simulink model "model4"  (R2024b)
settings: Solver=FixedStepAuto  StartTime=0.0  StopTime=500  FixedStep=0.001  RelTol=1e-3  EnableMultiTasking=on
libraries: arduinolib x2
settings Model: ExtModeTrigDuration=2  Creator=USER  LastModifiedBy=USER
settings SolverCC: AutoInsertRateTranBlk=on
settings OptimizationCC: EnhancedBackFolding=on  PassReuseOutputArgsAs=Individual arguments  ZeroExternalMemoryAtStartup=off  ZeroInternalMemoryAtStartup=off  MaxStackSize=64  OptimizeBlockOrder=speed  DifferentSizesBufferReuse=on  OptimizationCustomize=off  EfficientTunableParamExpr=on
settings DebuggingCC: ParameterTunabilityLossMsg=error
settings HardwareCC: ProdBitPerInt=16  ProdBitPerPointer=16  ProdBitPerSizeT=16  ProdBitPerPtrDiffT=16  ProdLargestAtomicFloat=None  ProdWordSize=8  ProdHWDeviceType=Atmel->AVR
settings SFSimCC: MATLABDynamicMemAlloc=off
settings RTWCC: Description=Embedded Coder  SystemTargetFile=ert.tlc  HardwareBoard=Arduino Mega 2560  TemplateMakefile=ert_default_tmf  Toolchain=Arduino AVR  BuildConfiguration=Faster Runs
settings CodeAppCC: ForceParamTrailComments=on  IgnoreCustomStorageClasses=off  OperatorAnnotations=on  SimulinkDataObjDesc=on  SFDataObjDesc=on  InsertBlockDesc=on
settings ERTTargetCC: SupportContinuousTime=on  SupportVariableSizeSignals=on  ExtModeTransport=3  ExtModeStaticAlloc=on  ExtModeAutomaticAllocSize=off  ExtModeStaticAllocSize=2048  ExtModeMexFile=ext_xcp  ExtModeIntrfLevel=Level2 - Open  InlinedParameterPlacement=Hierarchical

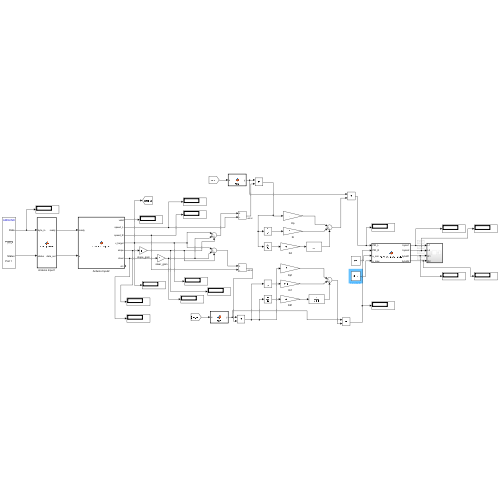
[thumbnail: Simulink's stored preview of the top-level diagram]
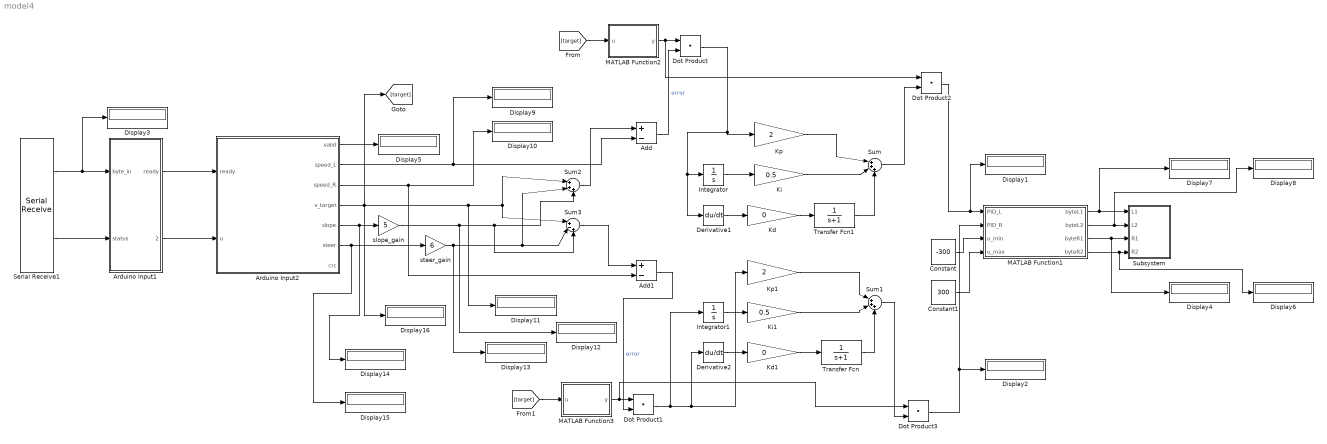
== system model4 ==
  Add : Sum  Inputs=+-  OutDataTypeStr=double  AccumDataTypeStr=double
  Add1 : Sum  Inputs=+-  OutDataTypeStr=double  AccumDataTypeStr=double
  Arduino Input1 : MATLAB Function  TreatAsAtomicUnit=on
  Arduino Input2 : MATLAB Function  TreatAsAtomicUnit=on
  Constant : Constant  Value=-300
  Constant1 : Constant  Value=300
  Derivative1 : Derivative
  Derivative2 : Derivative
  Display{1..16} (16 alike) : Display
      Display1 settings: Format=decimal (Stored Integer)
      Display10 settings: Format=decimal (Stored Integer)
      Display11 settings: Format=decimal (Stored Integer)
      Display13 settings: Format=decimal (Stored Integer)
      Display14 settings: Format=decimal (Stored Integer)
      Display15 settings: Format=decimal (Stored Integer)
      Display16 settings: Format=decimal (Stored Integer)
      Display2 settings: Format=decimal (Stored Integer)
      Display3 settings: Format=decimal (Stored Integer)
      Display4 settings: Format=decimal (Stored Integer)
      Display5 settings: Format=decimal (Stored Integer)
      Display6 settings: Format=decimal (Stored Integer)
      Display7 settings: Format=decimal (Stored Integer)
      Display8 settings: Format=decimal (Stored Integer)
      Display9 settings: Format=decimal (Stored Integer)
  Dot Product : DotProduct  OutDataTypeStr=Inherit: Inherit via internal rule
  Dot Product1 : DotProduct  OutDataTypeStr=Inherit: Inherit via internal rule
  Dot Product2 : DotProduct  OutDataTypeStr=int16
  Dot Product3 : DotProduct  OutDataTypeStr=int16
  Integrator : Integrator
  Integrator1 : Integrator
  Kd : Gain  Gain=0  ParamDataTypeStr=double  OutDataTypeStr=double
  Kd1 : Gain  Gain=0  ParamDataTypeStr=double  OutDataTypeStr=double
  Ki : Gain  Gain=0.5  ParamDataTypeStr=double  OutDataTypeStr=double
  Ki1 : Gain  Gain=0.5  ParamDataTypeStr=double  OutDataTypeStr=double
  Kp : Gain  Gain=2  ParamDataTypeStr=double  OutDataTypeStr=double
  Kp1 : Gain  Gain=2  ParamDataTypeStr=double  OutDataTypeStr=double
  MATLAB Function1 : MATLAB Function  TreatAsAtomicUnit=on
  MATLAB Function2 : MATLAB Function  TreatAsAtomicUnit=on
  MATLAB Function3 : MATLAB Function  TreatAsAtomicUnit=on
  Serial Receive1 : arduinolib/Serial Receive  portNumber=1  DataType=uint8  blockPlatform=ARDUINO  TimeOut=0  MaxDataLength=10  isARMArch=off  DataLengthOption=Length via dialog  Datalength=1  Header=[]  Terminator=[]  SampleTime=0.001  ShowOutStatus=on
      settings: SourceProductName=Common
  Subsystem : Subsystem  TreatAsAtomicUnit=on  SystemSampleTime=0.1
  Sum : Sum  Inputs=|+++  OutDataTypeStr=double
  Sum1 : Sum  Inputs=|+++  OutDataTypeStr=double
  Sum2 : Sum  Inputs=|+++  OutDataTypeStr=double  AccumDataTypeStr=double
  Sum3 : Sum  Inputs=|+-+  OutDataTypeStr=double  AccumDataTypeStr=double
  Transfer Fcn : TransferFcn  Denominator=[1 1]
  Transfer Fcn1 : TransferFcn  Denominator=[1 1]
  slope_gain : Gain  Gain=5
  steer_gain : Gain  Gain=6  ParamDataTypeStr=double  OutDataTypeStr=double
  wires:
  Arduino Input2/2(speed_L) -> Display9/1, Add/2
  Arduino Input2/4(v_target) -> [target], Display16/1, Display11/1, Sum2/1, Sum3/1
  Integrator/1 -> Ki/1
  Derivative1/1 -> Kd/1
  Kp/1 -> Sum/1
  Ki/1 -> Sum/2
  Kd/1 -> Transfer Fcn1/1
  Sum1/1 -> Dot Product3/2
  Arduino Input1/1(ready) -> Arduino Input2/1(ready)
  Serial Receive1/2 -> Arduino Input1/2(status)
  Arduino Input1/2(data_out) -> Arduino Input2/2(u)
  Serial Receive1/1 -> Display3/1, Arduino Input1/1(byte_in)
  Arduino Input2/3(speed_R) -> Add1/2, Display10/1
  Arduino Input2/1(valid) -> Display5/1
  Arduino Input2/6(steer) -> Display15/1, steer_gain/1
  steer_gain/1 -> Display13/1, Sum2/2, Sum3/2
  Sum2/1 -> Add/1
  Sum3/1 -> Add1/1
  Kd1/1 -> Transfer Fcn/1
  Ki1/1 -> Sum1/2
  Kp1/1 -> Sum1/1
  Derivative2/1 -> Kd1/1
  Integrator1/1 -> Ki1/1
  MATLAB Function1/2(byteL2) -> Display8/1, Subsystem/2(L2)
  MATLAB Function1/3(byteR1) -> Display4/1, Subsystem/3(R1)
  MATLAB Function1/4(byteR2) -> Display6/1, Subsystem/4(R2)
  Arduino Input2/5(slope) -> Display14/1, slope_gain/1
  slope_gain/1 -> Display12/1, Sum3/3, Sum2/3
  Transfer Fcn/1 -> Sum1/3
  Transfer Fcn1/1 -> Sum/3
  Sum/1 -> Dot Product2/2
  Constant/1 -> MATLAB Function1/3(u_min)
  Constant1/1 -> MATLAB Function1/4(u_max)
  MATLAB Function1/1(byteL1) -> Display7/1, Subsystem/1(L1)
  [target] -> MATLAB Function2/1(u)
  [target] -> MATLAB Function3/1(u)
  Add/1 -> Dot Product/2  "error"
  Dot Product/1 -> Derivative1/1, Integrator/1, Kp/1
  Add1/1 -> Dot Product1/2  "error"
  Dot Product1/1 -> Integrator1/1, Derivative2/1, Kp1/1
  MATLAB Function2/1(y) -> Dot Product2/1, Dot Product/1
  MATLAB Function3/1(y) -> Dot Product3/1, Dot Product1/1
  Dot Product3/1 -> MATLAB Function1/2(PID_R), Display2/1
  Dot Product2/1 -> Display1/1, MATLAB Function1/1(PID_L)

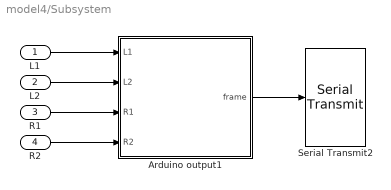
== system model4/Subsystem ==
  L1 : Inport
  L2 : Inport  Port=2
  R1 : Inport  Port=3
  R2 : Inport  Port=4
  Arduino output1 : MATLAB Function  TreatAsAtomicUnit=on
  Serial Transmit2 : arduinolib/Serial Transmit  portNumber=1  sendmode=write  sendformat=Decimal  floatprecision=2  header=[0xAA]  terminator=[0x55]  blockPlatform=ARDUINO
      settings: SourceProductName=Common
  wires:
  L2/1 -> Arduino output1/2(L2)
  Arduino output1/1(frame) -> Serial Transmit2/1
  L1/1 -> Arduino output1/1(L1)
  R1/1 -> Arduino output1/3(R1)
  R2/1 -> Arduino output1/4(R2)

== matlab function model4/MATLAB Function1 ==
  data: PID_L input; byteL1 output uint8; PID_R input; u_min input; u_max input; byteL2 output uint8; byteR1 output uint8; byteR2 output uint8
function [byteL1, byteL2, byteR1, byteR2] = encode_pwm_duty(PID_L, PID_R, u_min, u_max)
%#codegen

% [-1000, 1000] 범위로 선형 매핑
scale = 1000 / (u_max - u_min);
dutyL = int16(round((PID_L - u_min) * scale - 500));
dutyR = int16(round((PID_R - u_min) * scale - 500));

% uint16로 안전 변환 (비트 연산 위해)
dutyL_u = uint16(typecast(dutyL, 'uint16'));
dutyL_u = dutyL_u(1);
dutyR_u = uint16(typecast(dutyR, 'uint16'));
dutyR_u = dutyR_u(1);
% MSB / LSB 분리
byteL1 = uint8(bitshift(dutyL_u, -8));  % MSB
byteL2 = uint8(bitand(dutyL_u, 255));   % LSB

byteR1 = uint8(bitshift(dutyR_u, -8));
byteR2 = uint8(bitand(dutyR_u, 255));

% function [byteL1, byteL2, byteR1, byteR2] = encode_pwm_duty(PID_L, PID_R, u_min, u_max)
% % PID_L, PID_R : PID 제어기 출력값 (실수형)
% % u_min, u_max : PID 출력 예상 범위 (예: -4050 ~ +4050)
% 
% % 매핑 대상 범위
% min_duty = -1000;
% max_duty = 1000;
% 
% %% 매핑 함수 정의
% map_to_range = @(u) ((u - u_min) / (u_max - u_min)) * (max_duty - min_duty) + min_duty;
% 
% % 매핑 수행
% dutyL = int16(round(map_to_range(PID_L)));  % 정수로 변환
% dutyR = int16(round(map_to_range(PID_R)));
% 
% % MSB/LSB 분리
% byteL2 = bitand(dutyL, 255);         % LSB
% byteL1 = bitshift(dutyL, -8);        % MSB
% 
% byteR2 = bitand(dutyR, 255);
% byteR1 = bitshift(dutyR, -8);

== matlab function model4/MATLAB Function2 ==
  data: u input; y output
function y = fcn(u)

if u<1 && u > -1
    y=0;
else
    y=1;
end

== matlab function model4/Arduino Input2 ==
  data: ready input; valid output; speed_L output; speed_R output; v_target output; u input; slope output; steer output; crc output
function [valid, speed_L, speed_R, v_target, slope, steer, crc] =  Arduino_Input2( ready, u)
% UART 패킷 파서 (persistent 방식으로 이전 값 유지)
% u: [10x1] uint8, 패킷 데이터
% ready: 패킷 유효 신호

%#codegen

% 이전 출력값 저장용 persistent 변수
persistent p_valid p_speed_L p_speed_R p_v_target p_slope p_steer p_crc
 
% 초기화 (최초 실행 시)
if isempty(p_valid)
    p_valid = false;
    p_speed_L = 0.0;
    p_speed_R = 0.0;
    p_v_target = uint16(0);
    p_slope = int8(0);
    p_steer = int8(0);
    p_crc = uint8(0);
end

% 새로운 데이터가 들어왔을 경우만 업데이트
if ready == 1
    % data_sum = uint16((2)) + uint16(u(3)) + uint16(u(4)) + uint16(u(5)) + uint16(u(6)) + uint16(u(7)) + uint16(u(8)) + uint16(u(9));
    % if (0xFF & data_sum) == 0
        p_valid = true;
        p_speed_L = (double(u(2)-1) + double(u(3)-1)/100)*10;
        p_speed_R = (double(u(4)-1) + double(u(5)-1)/100)*10;
        if u(7)==1
            u(7)=u(7)-1;
        end
        p_v_target = uint16(u(7)-1)*10;
        tmp = typecast(u(6), 'int8'); tmp = tmp(1);
        if tmp <= int8(30) && tmp >= int8(-30)
            p_slope = tmp;
        end
        tmp = typecast(u(8), 'int8'); tmp = tmp(1);
        if  tmp <= int8(30) && tmp >= int8(-30)
            p_steer = tmp;
        end
        p_crc = u(9);
    % end
end

% 항상 마지막 유효 출력 반환
valid     = p_valid;
speed_L   = p_speed_L;
speed_R   = p_speed_R;
v_target  = p_v_target;
slope     = p_slope;
steer     = p_steer;
crc       = p_crc;

== matlab function model4/Arduino Input1 ==
  data: ready output; data_out output; byte_in input; status input
function [ready, data_out] = uart_parser(byte_in, status)
% UART 프레임 수신기 (Start Byte = 0xAA, Total = 10 bytes)
% 입력: byte_in - 1바이트씩 들어오는 uint8
% 입력: status - Serial Receive의 상태 (1이면 수신 성공)
% 출력: ready - 1이면 패킷 파싱 완료
% 출력: data_out - [1x10] uint8, 패킷 데이터

persistent buffer count collecting

if isempty(buffer)
    buffer = zeros(1, 10, 'uint8');
    count = 0;
    collecting = false;
end

ready = false;
data_out = zeros(1,10,'uint8');

if status == 1
    if ~collecting
        % 아직 수집 시작 전 → start byte 찾기
        if byte_in == hex2dec('AA')
            buffer(1) = byte_in;
            count = 1;
            collecting = true;
        end
    else
        if byte_in == hex2dec('AA')
            count = 1;
        end
        % 수집 중
        count = count + 1;
        buffer(count) = byte_in;

        if count == 10
            data_out = buffer;
            ready = true;
            count = 0;
            collecting = false;
        end
    end
else
    % if count~=0
    %     count = count + 1;
    %     buffer(count) = uint8(0);
    %     if count == 10
    %         data_out = buffer;
    %         ready = true;
    %         count = 0;
    %         collecting = false;
    %     end
    % else
        buffer = zeros(1, 10, 'uint8');
        count = 0;
        collecting = false;
    % end
end

== matlab function model4/MATLAB Function3 ==
  data: u input; y output
function y = fcn(u)

if u<1 && u > -1
    y=0;
else
    y=1;
end

== matlab function model4/Subsystem/Arduino output1 ==
  data: frame output; L1 input; L2 input; R1 input; R2 input
function frame = makeFrame(L1,L2,R1,R2)
% 입력:
%   vL, vR : 좌/우 목표 속도 (실수, cm/s 단위)
% 출력:
%   frame : 7-byte UART 전송 프레임 (uint8 벡터)
    frame = zeros(5,1,'uint8');  % 7바이트 프레임

    % 2-3. 목표속도_L (정수 + 소수)
    frame(1) = uint8(L1);                       % 정수부
    frame(2) = uint8(L2);       % 소수부 (소수점 둘째 자리까지)

    % 4-5. 목표속도_R (정수 + 소수)
    frame(3) = uint8(R1);                       % 정수부
    frame(4) = uint8(R2);       % 소수부

    % 6. CRC: 256 - (sum of byte 1~5) % 256
    crc = mod(sum(double(frame(1:5))), 256);
    frame(5) = uint8(mod(256 - crc, 256));
    
end
